simulink model "ProcessModelNonLin"  (R2019b)
settings: Solver=VariableStepAuto  StartTime=0.0  StopTime=10  RelTol=1e-3
settings Model: Creator=Daniel  LastModifiedBy=Daniel
settings DebuggingCC: UnderSpecifiedDimensionMsg=warning

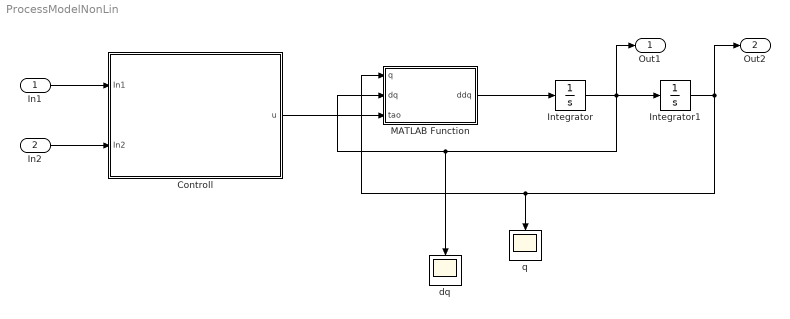
== system ProcessModelNonLin ==
  In1 : Inport
  In2 : Inport  Port=2
  Controll : Subsystem
  Integrator : Integrator  InitialCondition=[0;pi/6]
  Integrator1 : Integrator  InitialCondition=[0;0]
  MATLAB Function : MATLAB Function  TreatAsAtomicUnit=on
  dq : Scope
  q : Scope
  Out1 : Outport
  Out2 : Outport  Port=2
  wires:
  Integrator/1 -> Out1/1, dq/1, MATLAB Function/2(dq), Integrator1/1
  Integrator1/1 -> Out2/1, MATLAB Function/1(q), q/1
  Controll/1(u) -> MATLAB Function/3(tao)
  MATLAB Function/1(ddq) -> Integrator/1
  In1/1 -> Controll/1(In1)
  In2/1 -> Controll/2(In2)

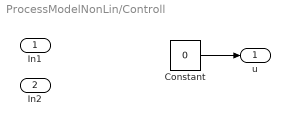
== system ProcessModelNonLin/Controll ==
  In1 : Inport
  In2 : Inport  Port=2
  Constant : Constant  Value=0
  u : Outport
  wires:
  Constant/1 -> u/1

== matlab function ProcessModelNonLin/MATLAB Function ==
  data: q input; ddq output; dq input; tao input
function  ddq  = testing(q,dq,tao)
%% q= [phi, theta],   dq = [dphi, dtheta]
tao2=[0;tao];
theta = q(2,1);
dtheta = dq(2,1);
dphi = dq(1,1);
%Given parameters - "competition.pdf"
la  = 75*10^-3;       %[m]      - Length of arm
r  = 43*10^-3;       %[m]      - Base radius
lp  = 31.5*10^-3;     %[m]      - Length of pendulum
J  = 125*10^-6;      %[kgm^2]  - Base moment of inertia
g  = 9.8;            %[m/s^2]  - Gravity
Jc = 2.55*10^-6;     %[kgm^2]  - Moment of inertia of pendulum around c.o.m
M  = 5.44*10^-3;     %[kg]     - Mass of pendulum point mass
Jp = 7.95*10^-6;     %[kgm^2]  - Moment of inertia of pend around pivot

%Still unknown - Try to guess these as a first step
ma = 10*10^-3;       %[kg] - Mass of arm       - Try 10g
mp = 5*10^-3;        %[kg] - Mass of pendulum  - Try 5g

%Equation (17)
alpha   = J + (M + (1/3)*ma + mp)*la^2;
beta    = (M + (1/3)*mp)*lp^2;
gamma   = (M + (1/2)*mp)*la*lp;
delta   = (M + (1/2)*mp)*g*lp;

D = [(alpha + beta*sin(theta)^2),(gamma*cos(theta));(gamma*cos(theta)),(beta)];
C = [(beta*cos(theta)*sin(theta)*dtheta),(beta*cos(theta)*sin(theta)*dphi - gamma*sin(theta)*dtheta);(-beta*cos(theta)*sin(theta)*dphi),(0)];
G = [0;-delta*sin(theta)];

% ddq = inv(D)*(tao2 - C*dq - G);
ddq = D\(tao2 - C*dq - G);
end
